simulink model "DC_motor_simulink"  (R2023b)
settings: Solver=VariableStepAuto  StartTime=0.0  StopTime=15  RelTol=1e-12
values from neighbouring files (symbols this model uses):
  A = [0   1 ... (first row only)    [DC_motor_example_LQR_v2.m]    (also in inverted_pendulum_main.m = [ 0         0               1                   0)
  B = [0 ... (first row only)    [DC_motor_example_LQR_v2.m]    (also in inverted_pendulum_main.m = [       0)
  K = lqr(A,B,Q,R)    [DC_motor_example_LQR_v2.m]    (also in inverted_pendulum_main.m = lqr(sys, Qf, Rf))
settings Model: Creator=magudelo  LastModifiedBy=loicdewit
settings SolverCC: AlgebraicLoopSolver=TrustRegion
settings OptimizationCC: LifeSpan=inf
settings DebuggingCC: UnconnectedInputMsg=warning  UnconnectedOutputMsg=warning  UnconnectedLineMsg=warning  SFExecutionAtInitializationDiag=none  ArithmeticOperatorsInVariantConditions=warning
settings ModelReferenceCC: EnableRefExpFcnMdlSchedulingChecks=on
settings SFSimCC: CustomCodeUndefinedFunction=UseInterfaceOnly
settings CodeAppCC: StateflowObjectComments=on

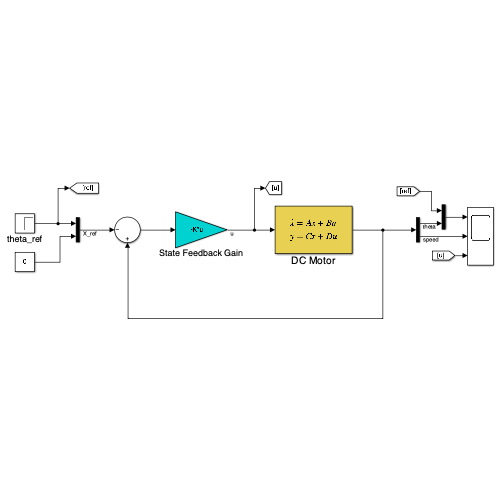
[thumbnail: Simulink's stored preview of the top-level diagram]
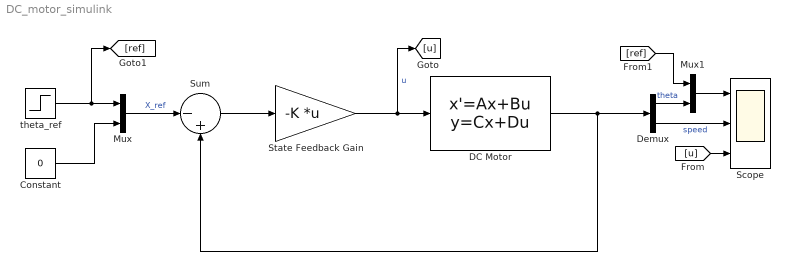
== system DC_motor_simulink ==
  Constant : Constant  Value=0
  DC Motor : StateSpace  A=A  B=B  C=eye(2,2)  D=zeros(2,1)  InitialCondition=0
  Demux : Demux  Outputs=2
  Mux : Mux  Inputs=2
  Mux1 : Mux  Inputs=2
  Scope : Scope  NumInputPorts=3
  State Feedback Gain : Gain  Gain=-K  Multiplication=Matrix(K*u)
  Sum : Sum  Inputs=|-+
  theta_ref : Step  SampleTime=0
  wires:
  Mux/1 -> Sum/1  "X_ref"
  Constant/1 -> Mux/2
  theta_ref/1 -> [ref], Mux/1
  Sum/1 -> State Feedback Gain/1
  State Feedback Gain/1 -> [u], DC Motor/1  "u"
  Demux/1 -> Mux1/2  "theta"
  Mux1/1 -> Scope/1
  Demux/2 -> Scope/2  "speed"
  [u] -> Scope/3
  [ref] -> Mux1/1
  DC Motor/1 -> Demux/1, Sum/2
